simulink model "Fuchs_FDFR_Simulink"  (R2024a)
settings: Solver=ode4  StartTime=0.0  StopTime=300.0  FixedStep=0.02  RelTol=1e-3
settings Model: Creator=finnf  LastModifiedBy=finnf

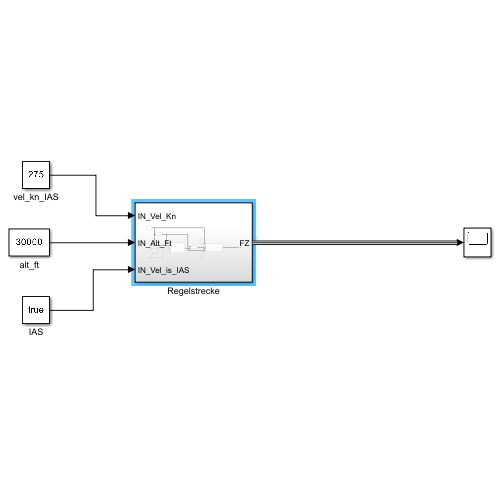
[thumbnail: Simulink's stored preview of the top-level diagram]
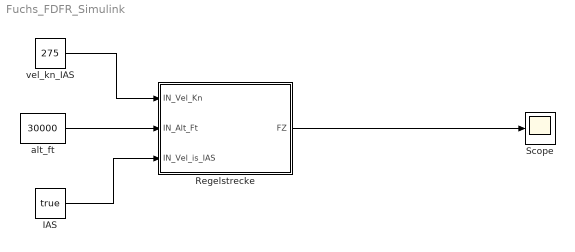
== system Fuchs_FDFR_Simulink ==
  IAS : Constant  Value=true
  Regelstrecke : Subsystem
  Scope : Scope
  alt_ft : Constant  Value=30000
  vel_kn_IAS : Constant  Value=275
  wires:
  vel_kn_IAS/1 -> Regelstrecke/1(IN_Vel_Kn)
  alt_ft/1 -> Regelstrecke/2(IN_Alt_Ft)
  IAS/1 -> Regelstrecke/3(IN_Vel_is_IAS)
  Regelstrecke/1(FZ) -> Scope/1

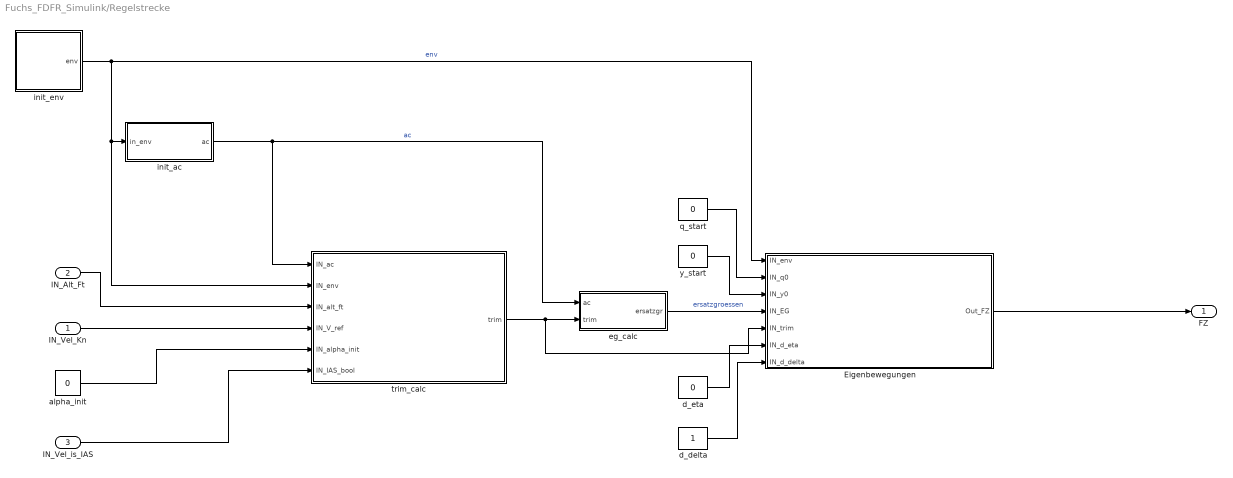
== system Fuchs_FDFR_Simulink/Regelstrecke ==
  IN_Vel_Kn : Inport
  IN_Alt_Ft : Inport  Port=2
  IN_Vel_is_IAS : Inport  Port=3
  Eigenbewegungen : Subsystem
  alpha_init : Constant  Value=0
  d_delta : Constant
  d_eta : Constant  Value=0
  eg_calc : Subsystem
  init_ac : Subsystem
  init_env : Subsystem
  q_start : Constant  Value=0
  trim_calc : Subsystem
  y_start : Constant  Value=0
  FZ : Outport
  wires:
  init_env/1(env) -> Eigenbewegungen/1(IN_env), trim_calc/2(IN_env), init_ac/1(in_env)  "env"
  init_ac/1(ac) -> eg_calc/1(ac), trim_calc/1(IN_ac)  "ac"
  trim_calc/1(trim) -> Eigenbewegungen/5(IN_trim), eg_calc/2(trim)
  IN_Alt_Ft/1 -> trim_calc/3(IN_alt_ft)
  IN_Vel_Kn/1 -> trim_calc/4(IN_V_ref)
  alpha_init/1 -> trim_calc/5(IN_alpha_init)
  IN_Vel_is_IAS/1 -> trim_calc/6(IN_IAS_bool)
  eg_calc/1(ersatzgr) -> Eigenbewegungen/4(IN_EG)  "ersatzgroessen"
  Eigenbewegungen/1(Out_FZ) -> FZ/1
  q_start/1 -> Eigenbewegungen/2(IN_q0)
  d_eta/1 -> Eigenbewegungen/6(IN_d_eta)
  d_delta/1 -> Eigenbewegungen/7(IN_d_delta)
  y_start/1 -> Eigenbewegungen/3(IN_y0)

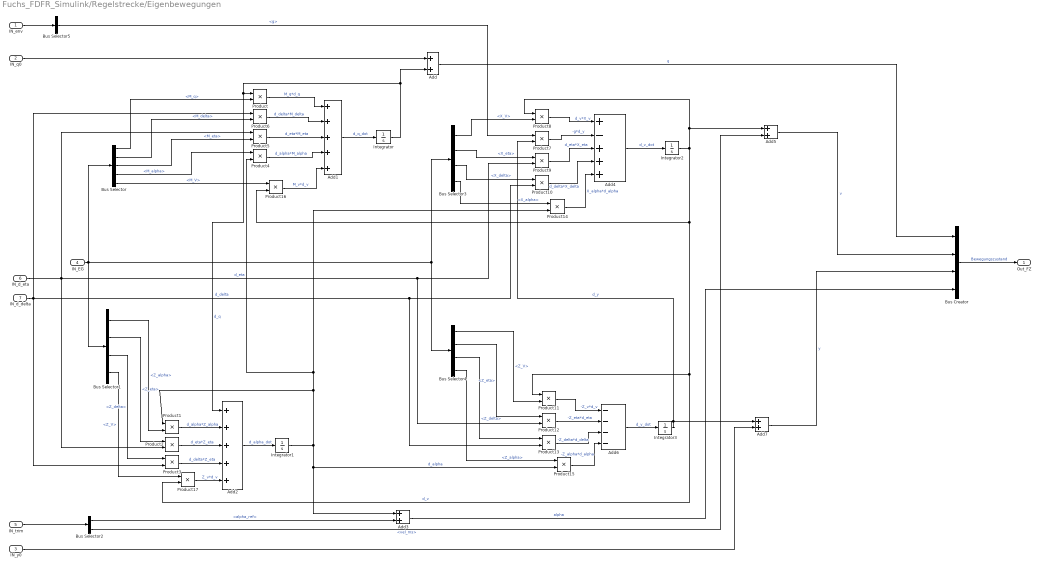
== system Fuchs_FDFR_Simulink/Regelstrecke/Eigenbewegungen ==
  IN_env : Inport
  IN_q0 : Inport  Port=2
  IN_y0 : Inport  Port=3
  IN_EG : Inport  Port=4
  IN_trim : Inport  Port=5
  IN_d_eta : Inport  Port=6
  IN_d_delta : Inport  Port=7
  Add{,3,5,7} (4 alike) : Sum
  Add1 : Sum  Inputs=+++++
  Add2 : Sum  Inputs=+++++
  Add4 : Sum  Inputs=+-+++
  Add6 : Sum  Inputs=----
  Bus Creator : BusCreator  Inputs=4
  Bus Selector : BusSelector  OutputSignals=M_q,M_delta,M_eta,M_alpha,M_V
  Bus Selector1 : BusSelector  OutputSignals=Z_alpha,Z_eta,Z_delta,Z_V
  Bus Selector2 : BusSelector  OutputSignals=alpha_ref,vel_ms
  Bus Selector3 : BusSelector  OutputSignals=X_V,X_eta,X_delta,X_alpha
  Bus Selector4 : BusSelector  OutputSignals=Z_V,Z_eta,Z_delta,Z_alpha
  Bus Selector5 : BusSelector  OutputSignals=g
  Integrator{,1..3} (4 alike) : Integrator
  Product{,1..17} (18 alike) : Product
  Out_FZ : Outport
  wires:
  IN_EG/1 -> Bus Selector4/1, Bus Selector3/1, Bus Selector1/1, Bus Selector/1
  Integrator/1 -> Add2/1, Product/1, Add/2  "d_q"
  Add1/1 -> Integrator/1  "d_q_dot"
  Bus Selector/1 -> Product/2  "<M_q>"
  Add2/1 -> Integrator1/1  "d_alpha_dot"
  Integrator1/1 -> Product14/2, Product4/2, Product1/1, Add3/1, Product15/2  "d_alpha"
  Bus Selector1/1 -> Product1/2  "<Z_alpha>"
  Product1/1 -> Add2/2  "d_alpha*Z_alpha"
  Bus Selector1/2 -> Product2/1  "<Z_eta>"
  IN_d_eta/1 -> Product2/2, Product12/2, Product9/2, Product5/1  "d_eta"
  Product2/1 -> Add2/3  "d_eta*Z_eta"
  Bus Selector1/3 -> Product3/1  "<Z_delta>"
  IN_d_delta/1 -> Product13/2, Product10/2, Product3/2, Product6/1  "d_delta"
  Product3/1 -> Add2/4  "d_delta*Z_eta"
  IN_trim/1 -> Bus Selector2/1
  Bus Selector2/1 -> Add3/2  "<alpha_ref>"
  IN_q0/1 -> Add/1
  Add/1 -> Bus Creator/1  "q"
  Bus Selector/4 -> Product4/1  "<M_alpha>"
  Product4/1 -> Add1/4  "d_alpha*M_alpha"
  Product/1 -> Add1/1  "M_q*d_q"
  Bus Selector/3 -> Product5/2  "<M_eta>"
  Product5/1 -> Add1/3  "d_eta*M_eta"
  Bus Selector/2 -> Product6/2  "<M_delta>"
  Product6/1 -> Add1/2  "d_delta*M_delta"
  Add3/1 -> Bus Creator/4  "alpha"
  Bus Creator/1 -> Out_FZ/1  "Bewegungszustand"
  IN_env/1 -> Bus Selector5/1
  Bus Selector5/1 -> Product7/1  "<g>"
  Product7/1 -> Add4/2  "-g*d_y"
  Add4/1 -> Integrator2/1  "d_v_dot"
  Integrator2/1 -> Product8/1, Add5/1, Product16/2, Product11/1, Product17/2  "d_v"
  Product8/1 -> Add4/1  "d_v*X_v"
  Bus Selector3/1 -> Product8/2  "<X_V>"
  Bus Selector3/2 -> Product9/1  "<X_eta>"
  Product9/1 -> Add4/3  "d_eta*X_eta"
  Bus Selector3/3 -> Product10/1  "<X_delta>"
  Product10/1 -> Add4/4  "d_delta*X_delta"
  Bus Selector2/2 -> Add5/2  "<vel_ms>"
  Add5/1 -> Bus Creator/2  "v"
  Add6/1 -> Integrator3/1  "d_y_dot"
  Integrator3/1 -> Add7/1, Product7/2  "d_y"
  Product11/1 -> Add6/1  "-Z_v*d_v"
  Bus Selector4/1 -> Product11/2  "<Z_V>"
  Bus Selector4/2 -> Product12/1  "<Z_eta>"
  Product12/1 -> Add6/2  "-Z_eta*d_eta"
  Product13/1 -> Add6/3  "-Z_delta*d_delta"
  IN_y0/1 -> Add7/2
  Add7/1 -> Bus Creator/3  "y"
  Product14/1 -> Add4/5  "X_alpha*d_alpha"
  Bus Selector3/4 -> Product14/1  "<X_alpha>"
  Bus Selector4/3 -> Product13/1  "<Z_delta>"
  Product15/1 -> Add6/4  "-Z_alpha*d_alpha"
  Bus Selector4/4 -> Product15/1  "<Z_alpha>"
  Product16/1 -> Add1/5  "M_v*d_v"
  Bus Selector/5 -> Product16/1  "<M_V>"
  Product17/1 -> Add2/5  "Z_v*d_v"
  Bus Selector1/4 -> Product17/1  "<Z_V>"

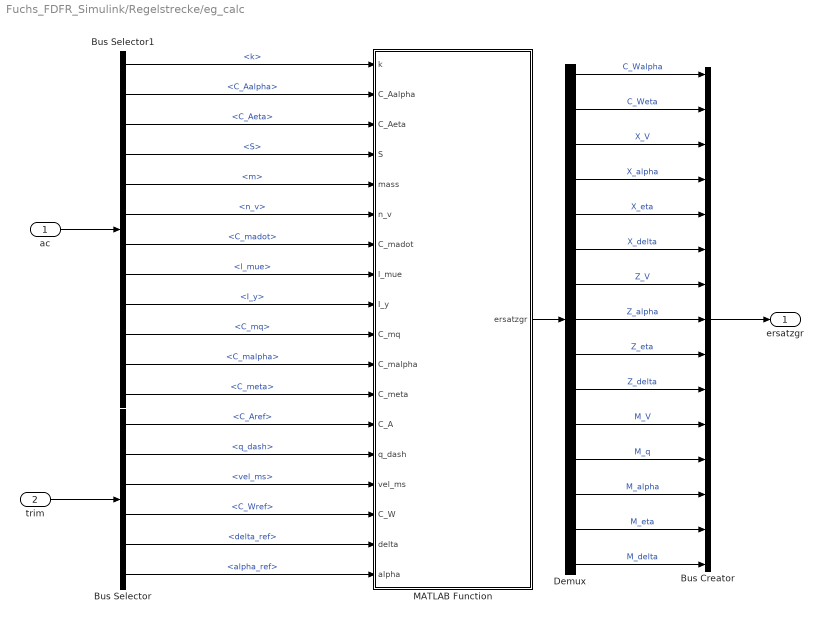
== system Fuchs_FDFR_Simulink/Regelstrecke/eg_calc ==
  ac : Inport
  trim : Inport  Port=2
  Bus Creator : BusCreator  Inputs=15
  Bus Selector : BusSelector  OutputSignals=C_Aref,q_dash,vel_ms,C_Wref,delta_ref,alpha_ref
  Bus Selector1 : BusSelector  OutputSignals=k,C_Aalpha,C_Aeta,S,m,n_v,C_madot,l_mue,I_y,C_mq,C_malpha,C_meta
  Demux : Demux  Outputs=15
  MATLAB Function : MATLAB Function  TreatAsAtomicUnit=on
  ersatzgr : Outport
  wires:
  trim/1 -> Bus Selector/1
  ac/1 -> Bus Selector1/1
  MATLAB Function/1(ersatzgr) -> Demux/1
  Bus Creator/1 -> ersatzgr/1
  Bus Selector1/1 -> MATLAB Function/1(k)  "<k>"
  Bus Selector1/2 -> MATLAB Function/2(C_Aalpha)  "<C_Aalpha>"
  Bus Selector1/3 -> MATLAB Function/3(C_Aeta)  "<C_Aeta>"
  Bus Selector1/4 -> MATLAB Function/4(S)  "<S>"
  Bus Selector1/5 -> MATLAB Function/5(mass)  "<m>"
  Bus Selector1/6 -> MATLAB Function/6(n_v)  "<n_v>"
  Bus Selector1/7 -> MATLAB Function/7(C_madot)  "<C_madot>"
  Bus Selector1/8 -> MATLAB Function/8(l_mue)  "<l_mue>"
  Bus Selector1/9 -> MATLAB Function/9(I_y)  "<I_y>"
  Bus Selector1/10 -> MATLAB Function/10(C_mq)  "<C_mq>"
  Bus Selector1/11 -> MATLAB Function/11(C_malpha)  "<C_malpha>"
  Bus Selector1/12 -> MATLAB Function/12(C_meta)  "<C_meta>"
  Bus Selector/1 -> MATLAB Function/13(C_A)  "<C_Aref>"
  Bus Selector/2 -> MATLAB Function/14(q_dash)  "<q_dash>"
  Bus Selector/3 -> MATLAB Function/15(vel_ms)  "<vel_ms>"
  Bus Selector/4 -> MATLAB Function/16(C_W)  "<C_Wref>"
  Bus Selector/5 -> MATLAB Function/17(delta)  "<delta_ref>"
  Bus Selector/6 -> MATLAB Function/18(alpha)  "<alpha_ref>"
  Demux/1 -> Bus Creator/1  "C_Walpha"
  Demux/2 -> Bus Creator/2  "C_Weta"
  Demux/3 -> Bus Creator/3  "X_V"
  Demux/4 -> Bus Creator/4  "X_alpha"
  Demux/5 -> Bus Creator/5  "X_eta"
  Demux/6 -> Bus Creator/6  "X_delta"
  Demux/7 -> Bus Creator/7  "Z_V"
  Demux/8 -> Bus Creator/8  "Z_alpha"
  Demux/9 -> Bus Creator/9  "Z_eta"
  Demux/10 -> Bus Creator/10  "Z_delta"
  Demux/11 -> Bus Creator/11  "M_V"
  Demux/12 -> Bus Creator/12  "M_q"
  Demux/13 -> Bus Creator/13  "M_alpha"
  Demux/14 -> Bus Creator/14  "M_eta"
  Demux/15 -> Bus Creator/15  "M_delta"

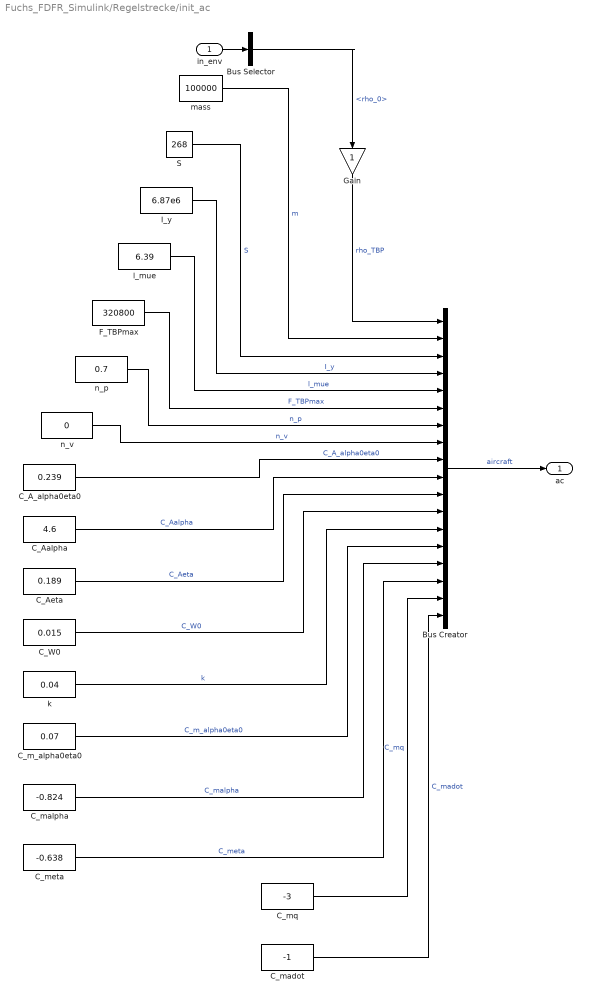
== system Fuchs_FDFR_Simulink/Regelstrecke/init_ac ==
  in_env : Inport
  Bus Creator : BusCreator  Inputs=18
  Bus Selector : BusSelector  OutputSignals=rho_0
  C_A_alpha0eta0 : Constant  Value=0.239
  C_Aalpha : Constant  Value=4.6
  C_Aeta : Constant  Value=0.189
  C_W0 : Constant  Value=0.015
  C_m_alpha0eta0 : Constant  Value=0.07
  C_madot : Constant  Value=-1
  C_malpha : Constant  Value=-0.824
  C_meta : Constant  Value=-0.638
  C_mq : Constant  Value=-3
  F_TBPmax : Constant  Value=320800
  Gain : Gain
  I_y : Constant  Value=6.87e6
  S : Constant  Value=268
  k : Constant  Value=0.04
  l_mue : Constant  Value=6.39
  mass : Constant  Value=100000
  n_p : Constant  Value=0.7
  n_v : Constant  Value=0
  ac : Outport
  wires:
  in_env/1 -> Bus Selector/1
  Bus Selector/1 -> Gain/1  "<rho_0>"
  Bus Creator/1 -> ac/1  "aircraft"
  mass/1 -> Bus Creator/2  "m"
  S/1 -> Bus Creator/3  "S"
  I_y/1 -> Bus Creator/4  "I_y"
  l_mue/1 -> Bus Creator/5  "l_mue"
  F_TBPmax/1 -> Bus Creator/6  "F_TBPmax"
  n_p/1 -> Bus Creator/7  "n_p"
  n_v/1 -> Bus Creator/8  "n_v"
  C_A_alpha0eta0/1 -> Bus Creator/9  "C_A_alpha0eta0"
  C_Aalpha/1 -> Bus Creator/10  "C_Aalpha"
  C_Aeta/1 -> Bus Creator/11  "C_Aeta"
  C_W0/1 -> Bus Creator/12  "C_W0"
  k/1 -> Bus Creator/13  "k"
  C_m_alpha0eta0/1 -> Bus Creator/14  "C_m_alpha0eta0"
  C_malpha/1 -> Bus Creator/15  "C_malpha"
  C_meta/1 -> Bus Creator/16  "C_meta"
  C_mq/1 -> Bus Creator/17  "C_mq"
  C_madot/1 -> Bus Creator/18  "C_madot"
  Gain/1 -> Bus Creator/1  "rho_TBP"

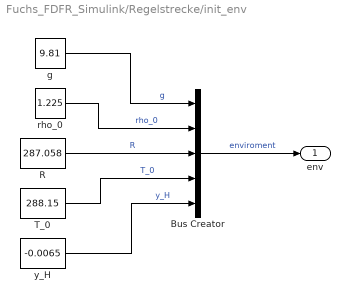
== system Fuchs_FDFR_Simulink/Regelstrecke/init_env ==
  Bus Creator : BusCreator  Inputs=5
  R : Constant  Value=287.058
  T_0 : Constant  Value=288.15
  g : Constant  Value=9.81
  rho_0 : Constant  Value=1.225
  y_H : Constant  Value=-0.0065
  env : Outport
  wires:
  Bus Creator/1 -> env/1  "enviroment"
  g/1 -> Bus Creator/1  "g"
  rho_0/1 -> Bus Creator/2  "rho_0"
  R/1 -> Bus Creator/3  "R"
  T_0/1 -> Bus Creator/4  "T_0"
  y_H/1 -> Bus Creator/5  "y_H"

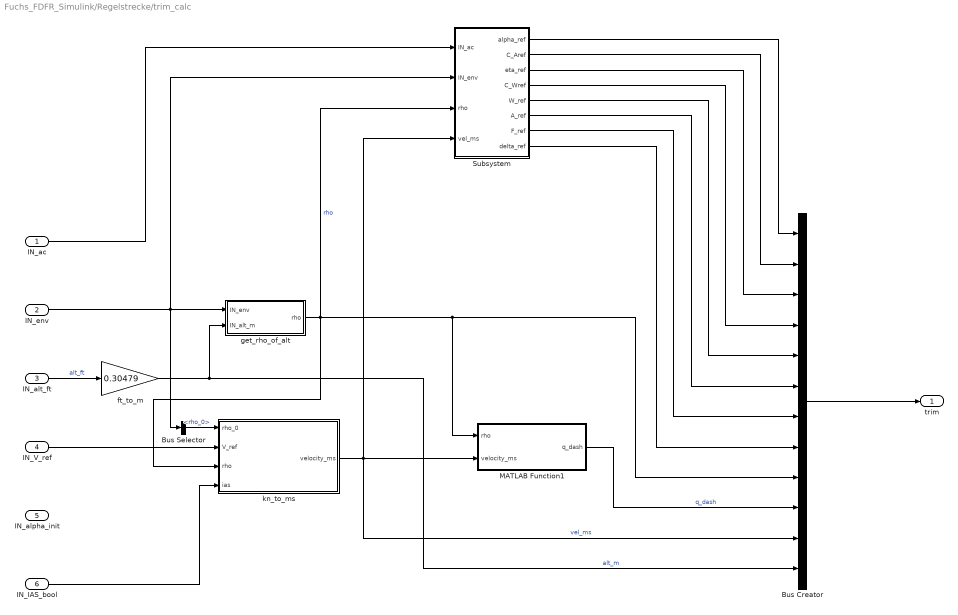
== system Fuchs_FDFR_Simulink/Regelstrecke/trim_calc ==
  IN_ac : Inport
  IN_env : Inport  Port=2
  IN_alt_ft : Inport  Port=3
  IN_V_ref : Inport  Port=4
  IN_alpha_init : Inport  Port=5
  IN_IAS_bool : Inport  Port=6
  Bus Creator : BusCreator  Inputs=12
  Bus Selector : BusSelector  OutputSignals=rho_0
  MATLAB Function1 : MATLAB Function  TreatAsAtomicUnit=on
  Subsystem : Subsystem
  ft_to_m : Gain  Gain=0.30479
  get_rho_of_alt : Subsystem
  kn_to_ms : MATLAB Function  TreatAsAtomicUnit=on
  trim : Outport
  wires:
  IN_alt_ft/1 -> ft_to_m/1  "alt_ft"
  Bus Creator/1 -> trim/1
  ft_to_m/1 -> get_rho_of_alt/2(IN_alt_m), Bus Creator/12  "alt_m"
  IN_env/1 -> Subsystem/2(IN_env), get_rho_of_alt/1(IN_env), Bus Selector/1
  IN_V_ref/1 -> kn_to_ms/2(V_ref)
  Bus Selector/1 -> kn_to_ms/1(rho_0)  "<rho_0>"
  get_rho_of_alt/1(rho) -> Subsystem/3(rho), Bus Creator/9, MATLAB Function1/1(rho), kn_to_ms/3(rho)  "rho"
  IN_IAS_bool/1 -> kn_to_ms/4(ias)
  kn_to_ms/1(velocity_ms) -> Subsystem/4(vel_ms), MATLAB Function1/2(velocity_ms), Bus Creator/11  "vel_ms"
  MATLAB Function1/1(q_dash) -> Bus Creator/10  "q_dash"
  IN_ac/1 -> Subsystem/1(IN_ac)
  Subsystem/1(alpha_ref) -> Bus Creator/1
  Subsystem/2(C_Aref) -> Bus Creator/2
  Subsystem/3(eta_ref) -> Bus Creator/3
  Subsystem/4(C_Wref) -> Bus Creator/4
  Subsystem/5(W_ref) -> Bus Creator/5
  Subsystem/6(A_ref) -> Bus Creator/6
  Subsystem/7(F_ref) -> Bus Creator/7
  Subsystem/8(delta_ref) -> Bus Creator/8

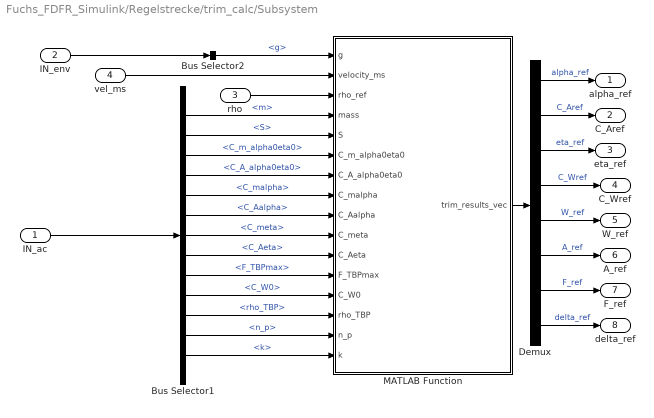
== system Fuchs_FDFR_Simulink/Regelstrecke/trim_calc/Subsystem ==
  IN_ac : Inport
  IN_env : Inport  Port=2
  rho : Inport  Port=3
  vel_ms : Inport  Port=4
  Bus Selector1 : BusSelector  OutputSignals=m,S,C_m_alpha0eta0,C_A_alpha0eta0,C_malpha,C_Aalpha,C_meta,C_Aeta,F_TBPmax,C_W0,rho_TBP,n_p,k
  Bus Selector2 : BusSelector  OutputSignals=g
  Demux : Demux  Outputs=8
  MATLAB Function : MATLAB Function  TreatAsAtomicUnit=on
  alpha_ref : Outport
  C_Aref : Outport  Port=2
  eta_ref : Outport  Port=3
  C_Wref : Outport  Port=4
  W_ref : Outport  Port=5
  A_ref : Outport  Port=6
  F_ref : Outport  Port=7
  delta_ref : Outport  Port=8
  wires:
  Bus Selector1/3 -> MATLAB Function/6(C_m_alpha0eta0)  "<C_m_alpha0eta0>"
  Bus Selector1/1 -> MATLAB Function/4(mass)  "<m>"
  Bus Selector1/12 -> MATLAB Function/15(n_p)  "<n_p>"
  Demux/1 -> alpha_ref/1  "alpha_ref"
  Bus Selector1/4 -> MATLAB Function/7(C_A_alpha0eta0)  "<C_A_alpha0eta0>"
  Bus Selector1/11 -> MATLAB Function/14(rho_TBP)  "<rho_TBP>"
  MATLAB Function/1(trim_results_vec) -> Demux/1
  Bus Selector1/8 -> MATLAB Function/11(C_Aeta)  "<C_Aeta>"
  Bus Selector1/5 -> MATLAB Function/8(C_malpha)  "<C_malpha>"
  Bus Selector1/10 -> MATLAB Function/13(C_W0)  "<C_W0>"
  Bus Selector1/6 -> MATLAB Function/9(C_Aalpha)  "<C_Aalpha>"
  Bus Selector1/9 -> MATLAB Function/12(F_TBPmax)  "<F_TBPmax>"
  Demux/8 -> delta_ref/1  "delta_ref"
  Bus Selector1/7 -> MATLAB Function/10(C_meta)  "<C_meta>"
  Bus Selector1/2 -> MATLAB Function/5(S)  "<S>"
  rho/1 -> MATLAB Function/3(rho_ref)
  Bus Selector2/1 -> MATLAB Function/1(g)  "<g>"
  Demux/6 -> A_ref/1  "A_ref"
  IN_env/1 -> Bus Selector2/1
  IN_ac/1 -> Bus Selector1/1
  Demux/4 -> C_Wref/1  "C_Wref"
  Demux/5 -> W_ref/1  "W_ref"
  Demux/3 -> eta_ref/1  "eta_ref"
  Demux/7 -> F_ref/1  "F_ref"
  vel_ms/1 -> MATLAB Function/2(velocity_ms)
  Demux/2 -> C_Aref/1  "C_Aref"
  Bus Selector1/13 -> MATLAB Function/16(k)  "<k>"

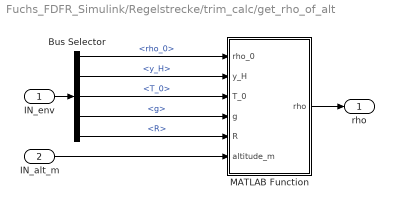
== system Fuchs_FDFR_Simulink/Regelstrecke/trim_calc/get_rho_of_alt ==
  IN_env : Inport
  IN_alt_m : Inport  Port=2
  Bus Selector : BusSelector  OutputSignals=rho_0,y_H,T_0,g,R
  MATLAB Function : MATLAB Function  TreatAsAtomicUnit=on
  rho : Outport
  wires:
  IN_alt_m/1 -> MATLAB Function/6(altitude_m)
  IN_env/1 -> Bus Selector/1
  Bus Selector/1 -> MATLAB Function/1(rho_0)  "<rho_0>"
  MATLAB Function/1(rho) -> rho/1
  Bus Selector/2 -> MATLAB Function/2(y_H)  "<y_H>"
  Bus Selector/3 -> MATLAB Function/3(T_0)  "<T_0>"
  Bus Selector/4 -> MATLAB Function/4(g)  "<g>"
  Bus Selector/5 -> MATLAB Function/5(R)  "<R>"

== matlab function Fuchs_FDFR_Simulink/Regelstrecke/trim_calc/kn_to_ms ==
  data: rho_0 input; V_ref input; velocity_ms output; rho input; ias input
function velocity_ms = fcn(rho_0, V_ref, rho, ias)
    if ias==false   %tas is given
            velocity_ms = (1852/3600) * V_ref;
        else            %ias is given
            velocity_ms = sqrt(rho_0/rho)*(1852/3600) * V_ref;
    end
end

== matlab function Fuchs_FDFR_Simulink/Regelstrecke/trim_calc/get_rho_of_alt/MATLAB Function ==
  data: rho_0 input; rho output; y_H input; T_0 input; g input; R input; altitude_m input
function rho = fcn(rho_0, y_H, T_0, g, R, altitude_m)
    rho = rho_0 * power((1+ (y_H/T_0)*altitude_m),(-(g/(R*y_H))-1));

== matlab function Fuchs_FDFR_Simulink/Regelstrecke/trim_calc/MATLAB Function1 ==
  data: rho input; q_dash output; velocity_ms input
function q_dash = fcn(rho, velocity_ms)
q_dash = (rho/2)*power(velocity_ms,2);

== matlab function Fuchs_FDFR_Simulink/Regelstrecke/trim_calc/Subsystem/MATLAB Function ==
  data: g input; velocity_ms input; rho_ref input; mass input; trim_results_vec output; S input; C_m_alpha0eta0 input; C_A_alpha0eta0 input; C_malpha input; C_Aalpha input; C_meta input; C_Aeta input; F_TBPmax input; C_W0 input; rho_TBP input; n_p input; k input
function trim_results_vec = fcn(g, velocity_ms ,rho_ref, mass, S, C_m_alpha0eta0, C_A_alpha0eta0, C_malpha, C_Aalpha, C_meta, C_Aeta, F_TBPmax, C_W0, rho_TBP, n_p, k)

    trim_results_vec = zeros(8,1);


    %does not change, so use as initial value
    C_Aref = (2*mass*g)/(rho_ref*power(velocity_ms,2)*S); % const

    %iteration
    for i=1:10
        eta_ref = -(C_m_alpha0eta0 + (C_Aref- C_A_alpha0eta0)*(C_malpha/C_Aalpha))/(C_meta - C_Aeta*(C_malpha/C_Aalpha));
        alpha_ref = (C_Aref - C_A_alpha0eta0 - C_Aeta*eta_ref)/C_Aalpha;
        
        C_Wref = C_W0 + k*power(C_Aref,2);
        W_ref = C_Wref*(rho_ref/2)*power(velocity_ms,2)*S;
        F_ref = W_ref / cos(alpha_ref);
        delta_ref = F_ref/(F_TBPmax*power(rho_ref/rho_TBP,n_p));

        A_ref = mass*g - F_ref*sin(alpha_ref);
        C_Aref = A_ref/((rho_ref/2)*power(velocity_ms,2)*S);
    end

    %reformat
    trim_results_vec(1) = alpha_ref;
    trim_results_vec(2) = C_Aref;
    trim_results_vec(3) = eta_ref;
    trim_results_vec(4) = C_Wref;
    trim_results_vec(5) = W_ref;
    trim_results_vec(6) = A_ref;
    trim_results_vec(7) = F_ref;
    trim_results_vec(8) = delta_ref;

== matlab function Fuchs_FDFR_Simulink/Regelstrecke/eg_calc/MATLAB Function ==
  data: k input; ersatzgr output; C_Aalpha input; C_Aeta input; S input; mass input; n_v input; C_madot input; l_mue input; I_y input; C_mq input; C_malpha input; C_meta input; C_A input; q_dash input; vel_ms input; C_W input; delta input; alpha input
function ersatzgr = fcn(k, C_Aalpha, C_Aeta, S, mass, n_v, C_madot, l_mue, I_y, C_mq, C_malpha, C_meta, C_A, q_dash, vel_ms, C_W, delta, alpha)
    ersatzgr = zeros(15,1);
    
    ersatzgr(1) = 2*k*C_A*C_Aalpha;
    ersatzgr(2) = 2*k*C_A*C_Aeta;
    
    ersatzgr(3) = -((q_dash*S)/(mass*vel_ms)*(2-n_v)*C_W);
    ersatzgr(4) = -((q_dash*S)/mass*ersatzgr(1));
    ersatzgr(5) = -((q_dash*S)/mass*ersatzgr(2));
    ersatzgr(6) = (q_dash*S)/mass*(C_W/delta);

    ersatzgr(7) = -2*((q_dash*S)/(mass*vel_ms)*(C_A/vel_ms));
    ersatzgr(8) = -((q_dash*S)/(mass*vel_ms)*C_Aalpha);
    ersatzgr(9) = -((q_dash*S)/(mass*vel_ms)*C_Aeta);
    ersatzgr(10) = - ersatzgr(6)*((tan(alpha))/vel_ms);

    ersatzgr(11) = ersatzgr(7) * ((q_dash*S*l_mue) / I_y) * (l_mue/vel_ms) * C_madot;
    ersatzgr(12) = ((q_dash*S*l_mue) / I_y) * (l_mue/vel_ms) * (C_mq + C_madot);
    ersatzgr(13) = ((q_dash*S*l_mue) / I_y) * (C_malpha + ersatzgr(8)*(l_mue/vel_ms)*C_madot);
    ersatzgr(14) = ((q_dash*S*l_mue) / I_y) * (C_meta + ersatzgr(9)*(l_mue/vel_ms)*C_madot);
    ersatzgr(15) = ersatzgr(10) * ((q_dash*S*l_mue) / I_y) * (l_mue/vel_ms) * C_madot;
